simulink model "CONVENTIONALtps30"  (Simulink 7.7)
settings: Solver=ode23t  SolverMode=SingleTasking  StartTime=0  StopTime=1.5  MaxStep=10e-6  RelTol=1e-4
libraries: powerlib x30, powerlib_extras x3, fuzblock x1
settings Model: Creator=patrice  LastModifiedBy=sabitha  ExtModeTrigMode=oneshot  ExtModeArmWhenConnect=off  ExtModeAutoUpdateStatusClock=off
settings DataIOCC: ExternalInput=[]  LimitDataPoints=off  SaveOutput=off  TimeSaveName=t  SignalLoggingName=sigsOut
settings OptimizationCC: BlockReduction=off  BooleanDataType=off  InlineInvariantSignals=on  InitFltsAndDblsToZero=on
settings DebuggingCC: SaveWithParameterizedLinksMsg=none  CheckExecutionContextPreStartOutputMsg=on  CheckExecutionContextRuntimeOutputMsg=on  SignalResolutionControl=TryResolveAllWithWarning  SolverPrmCheckMsg=none  MultiTaskDSMMsg=warning  MultiTaskCondExecSysMsg=none  SigSpecEnsureSampleTimeMsg=none  UnconnectedInputMsg=none  UnconnectedOutputMsg=none  StrictBusMsg=None
settings HardwareCC: TargetUnknown=on
settings RTWCC: IncludeERTFirstTime=on
settings GRTTargetCC: TargetFcnLib=ansi_tfl_tmw.mat

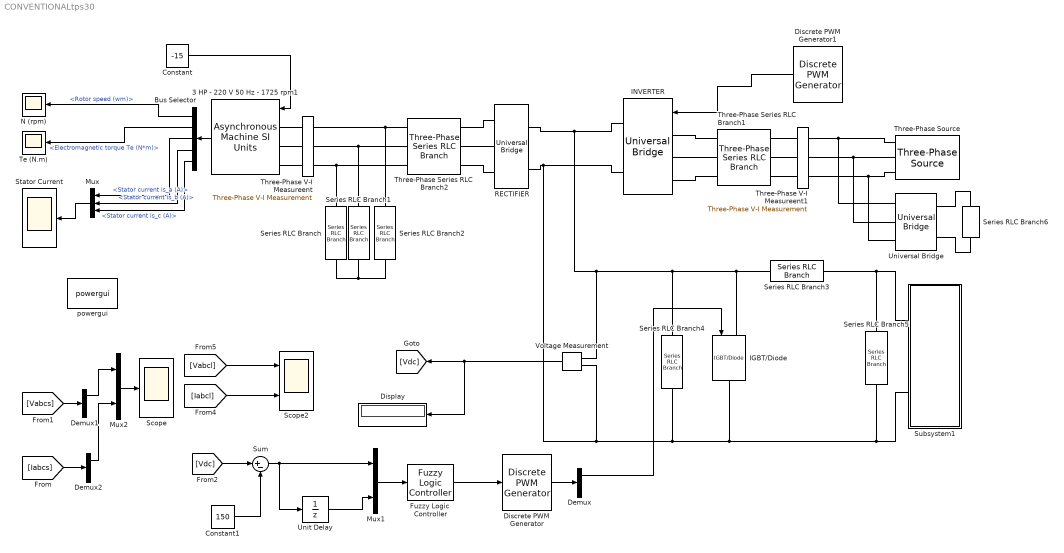
== system CONVENTIONALtps30 ==
  3 HP - 220 V 50 Hz - 1725 rpm1 : powerlib/Machines/Asynchronous Machine SI Units  SystemSampleTime=-1  PresetModel=No  MechanicalLoad=Torque Tm  ShowDetailedParameters=on  RotorType=Squirrel-cage  ReferenceFrame=Stationary  NominalParameters=[ 10*746, 230, 50 ]  Stator="[ 0.435  2*2.0e-3 ]"  Rotor="[ 0.816  2.0e-3 ]"  Cage1=[ 0.022 0.226/377]  Cage2=[ 0.022 0.226/377]  Lm=69.31e-3  Mechanical=[ 0.089 0 2 ]  PolePairs=2  InitialConditions="[ 1,0   0,0,0   0,0,0 ]"  Units=SI  LoadFlowParameters=0  SimulateSaturation=off  Saturation=[14.03593122, 27.81365428, 53.79336849, 72.68890987, 97.98006896, 148.6815601, 215.7428561, 302.9841135, 428.7778367 ; 230, 322, 414, 460, 506, 552, 598, 644, 690]  TsPowergui=0  TsBlock=-1  IterativeModel=Forward Euler  Pmec=0
  Bus Selector : BusSelector  OutputSignals=Mechanical.Rotor speed (wm),Mechanical.Electromagnetic torque Te (N*m),Stator measurements.Stator current is_a (A),Stator measurements.Stator current is_b (A),Stator measurements.Stator current is_c (A)
  Constant : Constant  Value=-15
  Constant1 : Constant  Value=150
  Demux : Demux  Outputs=2
  Demux1 : Demux  Outputs=3
  Demux2 : Demux  Outputs=3
  Discrete PWM Generator : powerlib_extras/Discrete  Control Blocks/Discrete PWM Generator  SystemSampleTime=-1  GeneratorMode="1-arm  bridge (2 pulses)"  Fc=1080  Ts=5e-6  Internal=off  mIndex=0.4  Freq=60  Phase=0
  Discrete PWM Generator1 : powerlib_extras/Discrete  Control Blocks/Discrete PWM Generator  SystemSampleTime=-1  GeneratorMode="3-arm  bridge (6 pulses)"  Fc=1080  Ts=5e-6  Internal=on  mIndex=0.4  Freq=60  Phase=0
  Display : Display
  Fuzzy Logic  Controller : fuzblock/Fuzzy Logic  Controller  SystemSampleTime=-1  fis=vienna_fuzzy
  IGBT/Diode : powerlib/Power Electronics/IGBT//Diode  SystemSampleTime=-1  Ron=1e-3  Rs=1e5  Cs=inf  Measurements=off
  INVERTER : powerlib/Power Electronics/Universal Bridge  SystemSampleTime=-1  Arms=3  SnubberResistance=1e5  SnubberCapacitance=inf  Device=IGBT / Diodes  Ron=12  Lon=0  ForwardVoltages="[  0  0  ]"  ForwardVoltage=0  GTOparameters=[ 10e-6 , 20e-6 ]  IGBTparameters=[ 1e-6 , 2e-6 ]  Measurements=None  Measurements_2=None  converterType=Rectifier
  Mux : Mux  Inputs=3
  Mux1 : Mux  Inputs=2
  Mux2 : Mux  Inputs=2
  N (rpm) : Scope
      settings: TimeRange=0.2  YMin=759  YMax=769  DataFormat=Structure
  RECTIFIER : powerlib/Power Electronics/Universal Bridge  SystemSampleTime=-1  Arms=3  SnubberResistance=1e5  SnubberCapacitance=inf  Device=Diodes  Ron=12  Lon=0  ForwardVoltages="[  0  0  ]"  ForwardVoltage=0  GTOparameters=[ 10e-6 , 20e-6 ]  IGBTparameters=[ 1e-6 , 2e-6 ]  Measurements=None  Measurements_2=None  converterType=Rectifier
  Scope : Scope
      settings: TimeRange=0.25  YMax=90  SaveName=rectifiersource
  Scope2 : Scope  NumInputPorts=2
      settings: TimeRange=1  YMin=-225~-6  YMax=225~8  SaveName=rectifierload
  Series RLC Branch : powerlib/Elements/Series RLC Branch  PhysicalDomain=powersysdomain  SubClassName=unknown  LeftPortType=p1  RightPortType=p1  LConnTagsString=__new0  RConnTagsString=__new0  BranchType=C  Resistance=1  Inductance=1e-3  SetiL0=off  InitialCurrent=0  Capacitance=3e-3  Setx0=off  InitialVoltage=0  Measurements=None
  Series RLC Branch1 : powerlib/Elements/Series RLC Branch  PhysicalDomain=powersysdomain  SubClassName=unknown  LeftPortType=p1  RightPortType=p1  LConnTagsString=__new0  RConnTagsString=__new0  BranchType=C  Resistance=1  Inductance=1e-3  SetiL0=off  InitialCurrent=0  Capacitance=3e-3  Setx0=off  InitialVoltage=0  Measurements=None
  Series RLC Branch2 : powerlib/Elements/Series RLC Branch  PhysicalDomain=powersysdomain  SubClassName=unknown  LeftPortType=p1  RightPortType=p1  LConnTagsString=__new0  RConnTagsString=__new0  BranchType=C  Resistance=1  Inductance=1e-3  SetiL0=off  InitialCurrent=0  Capacitance=3e-3  Setx0=off  InitialVoltage=0  Measurements=None
  Series RLC Branch3 : powerlib/Elements/Series RLC Branch  PhysicalDomain=powersysdomain  SubClassName=unknown  LeftPortType=p1  RightPortType=p1  LConnTagsString=__new0  RConnTagsString=__new0  BranchType=L  Resistance=1  Inductance=100e-3  SetiL0=off  InitialCurrent=0  Capacitance=1e-6  Setx0=off  InitialVoltage=0  Measurements=None
  Series RLC Branch4 : powerlib/Elements/Series RLC Branch  PhysicalDomain=powersysdomain  SubClassName=unknown  LeftPortType=p1  RightPortType=p1  LConnTagsString=__new0  RConnTagsString=__new0  BranchType=C  Resistance=1  Inductance=1e-3  SetiL0=off  InitialCurrent=0  Capacitance=10e-6  Setx0=off  InitialVoltage=0  Measurements=None
  Series RLC Branch5 : powerlib/Elements/Series RLC Branch  PhysicalDomain=powersysdomain  SubClassName=unknown  LeftPortType=p1  RightPortType=p1  LConnTagsString=__new0  RConnTagsString=__new0  BranchType=C  Resistance=1  Inductance=1e-3  SetiL0=off  InitialCurrent=0  Capacitance=1e-6  Setx0=off  InitialVoltage=0  Measurements=None
  Series RLC Branch6 : powerlib/Elements/Series RLC Branch  PhysicalDomain=powersysdomain  SubClassName=unknown  LeftPortType=p1  RightPortType=p1  LConnTagsString=__new0  RConnTagsString=__new0  BranchType=RL  Resistance=1  Inductance=1e-3  SetiL0=off  InitialCurrent=0  Capacitance=10e-6  Setx0=off  InitialVoltage=0  Measurements=None
  Stator Current : Scope
      settings: TimeRange=0.25  YMin=-0.6  YMax=0.7  SaveName=ScopeData7
  Subsystem1 : Subsystem
  Sum : Sum  Inputs=|+-
  Te (N.m) : Scope
      settings: YMin=-5.5e-023  YMax=-2e-023  DataFormat=Structure
  Three-Phase Series RLC Branch1 : powerlib/Elements/Three-Phase Series RLC Branch  PhysicalDomain=powersysdomain  SubClassName=unknown  LeftPortType=p1  RightPortType=p1  LConnTagsString=A|B|C  RConnTagsString=A|B|C  BranchType=RL  Resistance=0.1  Inductance=0.1  Capacitance=1e-6  Measurements=None
  Three-Phase Series RLC Branch2 : powerlib/Elements/Three-Phase Series RLC Branch  PhysicalDomain=powersysdomain  SubClassName=unknown  LeftPortType=p1  RightPortType=p1  LConnTagsString=A|B|C  RConnTagsString=A|B|C  BranchType=RL  Resistance=0.1  Inductance=1e-3  Capacitance=1e-6  Measurements=None
  Three-Phase V-I Measureent : powerlib/Measurements/Three-Phase V-I Measurement  SystemSampleTime=-1  VoltageMeasurement=phase-to-ground  SetLabelV=on  LabelV=Vabcs  Vpu=off  VpuLL=off  CurrentMeasurement=yes  SetLabelI=on  LabelI=Iabcs  Ipu=off  Pbase=100e6  Vbase=500e3  OutputType=Complex  PhasorSimulation=off  PSBequivalent=0
  Three-Phase V-I Measureent1 : powerlib/Measurements/Three-Phase V-I Measurement  SystemSampleTime=-1  VoltageMeasurement=phase-to-ground  SetLabelV=on  LabelV=Vabcl  Vpu=off  VpuLL=off  CurrentMeasurement=yes  SetLabelI=on  LabelI=Iabcl  Ipu=off  Pbase=100e6  Vbase=500e3  OutputType=Complex  PhasorSimulation=off  PSBequivalent=0
  Three-Phase Source : powerlib/Electrical Sources/Three-Phase Source  SystemSampleTime=-1  Voltage=230*sqrt(3/2)  PhaseAngle=0  Frequency=50  InternalConnection=Yg  SpecifyImpedance=on  Resistance=0.8929  Inductance=16.58e-3  ShortCircuitLevel=25e3  BaseVoltage=230*sqrt(3/2)  XRratio=7  BusType=swing  Pref=0  Qref=0  Qmin=-inf  Qmax=inf
  Unit Delay : UnitDelay  SampleTime=-1
  Universal Bridge : powerlib/Power Electronics/Universal Bridge  SystemSampleTime=-1  Arms=3  SnubberResistance=100  SnubberCapacitance=inf  Device=Diodes  Ron=1e-3  Lon=0  ForwardVoltages="[  0  0  ]"  ForwardVoltage=0  GTOparameters=[ 10e-6 , 20e-6 ]  IGBTparameters=[ 1e-6 , 2e-6 ]  Measurements=None  Measurements_2=None  converterType=Rectifier
  Voltage Measurement : powerlib/Measurements/Voltage Measurement  SystemSampleTime=-1  PhasorSimulation=off  OutputType=Complex  PSBequivalent=0
  powergui : powerlib/powergui  Priority=1  SystemSampleTime=-1  SimulationMode=Discrete  SampleTime=50e-6  frequency=60  SPID=off  DisableSnubberDevices=off  DisableRonSwitches=off  DisableVfSwitches=off  SwTol=0  Interpol=off  DisplayEquations=off  FunctionMessages=off  frequencyindice=0  Pbase=100e6  ErrMax=1e-4  Iterations=50  UnitsV=kV  UnitsW=MW  echomessages=off  HookPort=off  EnableUseOfTLC=off  x0status=blocks  RestoreLinks=warning  ResistiveCurrentMeasurement=off  Ylog=off  Xlog=on  ShowGrid=off  save=off  variable=ZData  structure=rectifierload  ZoomFFT=off  StartTime=1.4  cycles=1  DisplayStyle=1  fundamental=50  FreqAxis=off  MaxFrequency=1000  frequencyindicesteady=1  display=off  methode=off
  wires:
  [Vabcl] -> Scope2/1
  [Iabcl] -> Scope2/2
  Bus Selector/2 -> Te (N.m)/1  "<Electromagnetic torque Te (N*m)>"
  Constant/1 -> 3 HP - 220 V 50 Hz - 1725 rpm1/1
  Bus Selector/1 -> N (rpm)/1  "<Rotor speed (wm)>"
  3 HP - 220 V 50 Hz - 1725 rpm1/1 -> Bus Selector/1
  Bus Selector/3 -> Mux/1  "<Stator current is_a (A)>"
  Bus Selector/4 -> Mux/2  "<Stator current is_b (A)>"
  Bus Selector/5 -> Mux/3  "<Stator current is_c (A)>"
  Mux/1 -> Stator Current/1
  Discrete PWM Generator1/1 -> INVERTER/1
  Voltage Measurement/1 -> [Vdc], Display/1
  [Vdc] -> Sum/1
  Constant1/1 -> Sum/2
  Sum/1 -> Unit Delay/1, Mux1/1
  Unit Delay/1 -> Mux1/2
  Mux1/1 -> Fuzzy Logic  Controller/1
  Fuzzy Logic  Controller/1 -> Discrete PWM Generator/1
  Discrete PWM Generator/1 -> Demux/1
  Demux/1 -> IGBT/Diode/1
  Mux2/1 -> Scope/1
  [Vabcs] -> Demux1/1
  Demux1/1 -> Mux2/1
  [Iabcs] -> Demux2/1
  Demux2/1 -> Mux2/2
  connections:
  Three-Phase Series RLC Branch1/RConn1 -- Three-Phase V-I Measureent1/LConn1
  Three-Phase Series RLC Branch1/RConn2 -- Three-Phase V-I Measureent1/LConn2
  Three-Phase Series RLC Branch1/RConn3 -- Three-Phase V-I Measureent1/LConn3
  Series RLC Branch2/LConn1 -- Three-Phase V-I Measureent/RConn1 -- Three-Phase Series RLC Branch2/LConn1
  Series RLC Branch1/LConn1 -- Three-Phase V-I Measureent/RConn2 -- Three-Phase Series RLC Branch2/LConn2
  3 HP - 220 V 50 Hz - 1725 rpm1/LConn3 -- Three-Phase V-I Measureent/LConn3
  3 HP - 220 V 50 Hz - 1725 rpm1/LConn2 -- Three-Phase V-I Measureent/LConn2
  3 HP - 220 V 50 Hz - 1725 rpm1/LConn1 -- Three-Phase V-I Measureent/LConn1
  RECTIFIER/RConn2 -- IGBT/Diode/RConn1 -- Series RLC Branch5/RConn1 -- Subsystem1/LConn2 -- Series RLC Branch4/RConn1 -- Voltage Measurement/LConn2 -- INVERTER/RConn2
  INVERTER/LConn2 -- Three-Phase Series RLC Branch1/LConn2
  INVERTER/LConn1 -- Three-Phase Series RLC Branch1/LConn1
  INVERTER/LConn3 -- Three-Phase Series RLC Branch1/LConn3
  Series RLC Branch3/RConn1 -- Series RLC Branch5/LConn1 -- Subsystem1/LConn1
  Universal Bridge/LConn2 -- Three-Phase V-I Measureent1/RConn2 -- Three-Phase Source/RConn2
  Universal Bridge/LConn3 -- Three-Phase Source/RConn3 -- Three-Phase V-I Measureent1/RConn3
  Universal Bridge/LConn1 -- Three-Phase Source/RConn1 -- Three-Phase V-I Measureent1/RConn1
  RECTIFIER/RConn1 -- Series RLC Branch4/LConn1 -- IGBT/Diode/LConn1 -- Series RLC Branch3/LConn1 -- Voltage Measurement/LConn1 -- INVERTER/RConn1
  Series RLC Branch2/RConn1 -- Series RLC Branch/RConn1 -- Series RLC Branch1/RConn1
  Series RLC Branch/LConn1 -- Three-Phase V-I Measureent/RConn3 -- Three-Phase Series RLC Branch2/LConn3
  Three-Phase Series RLC Branch2/RConn2 -- RECTIFIER/LConn2
  Three-Phase Series RLC Branch2/RConn3 -- RECTIFIER/LConn3
  Three-Phase Series RLC Branch2/RConn1 -- RECTIFIER/LConn1
  Universal Bridge/RConn1 -- Series RLC Branch6/LConn1
  Universal Bridge/RConn2 -- Series RLC Branch6/RConn1

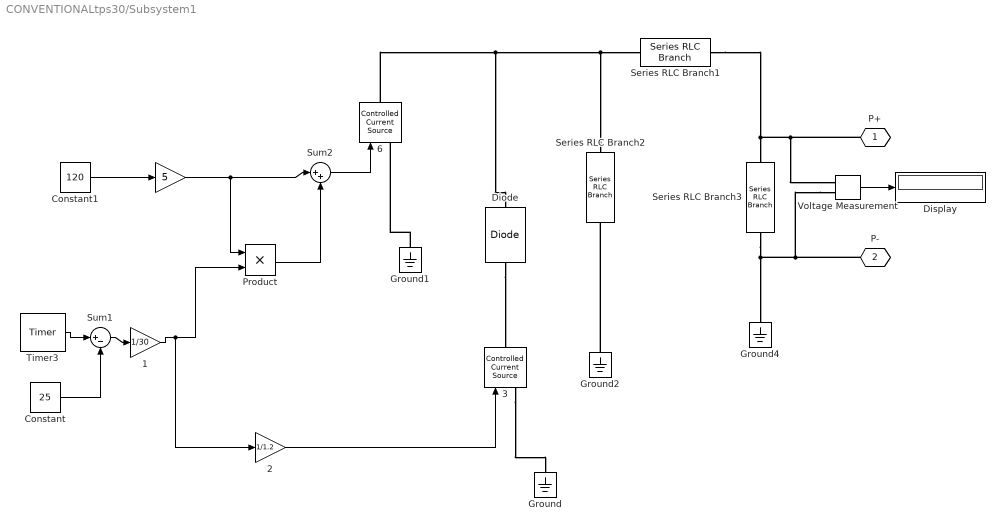
== system CONVENTIONALtps30/Subsystem1 ==
  "  " : Gain  Gain=5  OutDataTypeStr=Inherit: Inherit via back propagation  RndMeth=Zero
  "  1" : Gain  Gain=1/30  RndMeth=Zero
  "  2" : Gain  Gain=1/1.2  OutDataTypeStr=Inherit: Inherit via back propagation  RndMeth=Zero
  "  3" : powerlib/Electrical Sources/Controlled Current Source  Description=source block  SystemSampleTime=-1  Initialize=on  Source_Type=AC  Amplitude=0  Phase=0  Frequency=0  Measurements=None
      settings: AttributesFormatString=\n
  "  6" : powerlib/Electrical Sources/Controlled Current Source  Description=source block  SystemSampleTime=-1  Initialize=on  Source_Type=AC  Amplitude=0  Phase=0  Frequency=0  Measurements=None
      settings: AttributesFormatString=\n
  Constant : Constant  Value=25
  Constant1 : Constant  Value=120
  Diode : powerlib/Power Electronics/Diode  SystemSampleTime=-1  Ron=0.001  Lon=0  Vf=0.8  IC=0  UseSnubber=off  Rs=500  Cs=250e-9  Measurements=off
  Display : Display
  Ground{,1..2,4} (4 alike) : powerlib/Elements/Ground  PhysicalDomain=powersysdomain  SubClassName=unknown  LeftPortType=p1  RightPortType=p1  LConnTagsString=a
  Product : Product  SaturateOnIntegerOverflow=on  RndMeth=Zero  OutDataTypeStr=Inherit: Same as first input
  Series RLC Branch1 : powerlib/Elements/Series RLC Branch  PhysicalDomain=powersysdomain  SubClassName=unknown  LeftPortType=p1  RightPortType=p1  LConnTagsString=__new0  RConnTagsString=__new0  BranchType=R  Resistance=50  Inductance=1e-3  SetiL0=off  InitialCurrent=0  Capacitance=1e-6  Setx0=off  InitialVoltage=0  Measurements=None
  Series RLC Branch2 : powerlib/Elements/Series RLC Branch  PhysicalDomain=powersysdomain  SubClassName=unknown  LeftPortType=p1  RightPortType=p1  LConnTagsString=__new0  RConnTagsString=__new0  BranchType=R  Resistance=0.11  Inductance=1e-3  SetiL0=off  InitialCurrent=0  Capacitance=1e-6  Setx0=off  InitialVoltage=0  Measurements=None
  Series RLC Branch3 : powerlib/Elements/Series RLC Branch  PhysicalDomain=powersysdomain  SubClassName=unknown  LeftPortType=p1  RightPortType=p1  LConnTagsString=__new0  RConnTagsString=__new0  BranchType=R  Resistance=10  Inductance=1e-3  SetiL0=off  InitialCurrent=0  Capacitance=1e-6  Setx0=off  InitialVoltage=0  Measurements=None
  Sum1 : Sum  Inputs=|+-  SaturateOnIntegerOverflow=on
  Sum2 : Sum  Inputs=|++  SaturateOnIntegerOverflow=on
  Timer3 : powerlib_extras/Control  Blocks/Timer  SystemSampleTime=-1  t=0.001  e=200
  Voltage Measurement : powerlib/Measurements/Voltage Measurement  SystemSampleTime=-1  PhasorSimulation=off  OutputType=Complex  PSBequivalent=0
  P+ : PMIOPort  Tag=PMCPort  Port=1  Side=Left
  P- : PMIOPort  Tag=PMCPort  Port=2  Side=Left
  wires:
  Constant1/1 -> "  "/1
  Timer3/1 -> Sum1/1
  Product/1 -> Sum2/2
  "  "/1 -> Sum2/1, Product/1
  Sum2/1 -> "  6"/1
  "  2"/1 -> "  3"/1
  Constant/1 -> Sum1/2
  Sum1/1 -> "  1"/1
  "  1"/1 -> "  2"/1, Product/2
  Voltage Measurement/1 -> Display/1
  connections:
  Voltage Measurement/LConn2 -- Ground4/LConn1 -- Series RLC Branch3/RConn1 -- P-/RConn1
  Ground2/LConn1 -- Series RLC Branch2/RConn1
  Series RLC Branch1/RConn1 -- Voltage Measurement/LConn1 -- P+/RConn1 -- Series RLC Branch3/LConn1
  Diode/LConn1 -- Series RLC Branch1/LConn1 -- Series RLC Branch2/LConn1 -- "  6"/RConn1
  Ground1/LConn1 -- "  6"/LConn1
  Diode/RConn1 -- "  3"/RConn1
  "  3"/LConn1 -- Ground/LConn1
